simulink model "JenaFox_moodle_ISB"  (R2018a)
settings: Solver=ode23s  StartTime=0.0  StopTime=60  MaxStep=maxStep  RelTol=relTol  AbsTol=absTol
InitFcn:
  | Fox_param;
model workspace: external: MAT-File C:\Users\Work\Documents\MATLAB\JenaFoxSimulink\moodle model\simulink_robot_DataFile.mat (data not in the file)
undefined symbols (not defined in the file or in its folder): amplifier, c_coupling_hip, c_coupling_knee, c_hs, d_coupling_knee, d_hs, g, hip_i, hip_Jm, hip_k, hip_Mrg, hip_Mrhg, hip_na, hip_Ra, IC_motor_hip_l, IC_motor_hip_r, IC_motor_knee_l, IC_motor_knee_r, IC_phi_hip_l, IC_phi_hip_r, IC_v_motor_hip, IC_v_motor_knee, k_gx, k_gy, knee_i, knee_Jm, knee_k, knee_Mrg, knee_Mrhg, knee_na, knee_Ra, mu_slide, mu_stick, smiData, v_gx_max, v_gy_max, vLimit, X, Y, Z
libraries: sm_lib x38, nesl_utility x28, simulink x22, simulink_extras x8
(part 3 of 3)

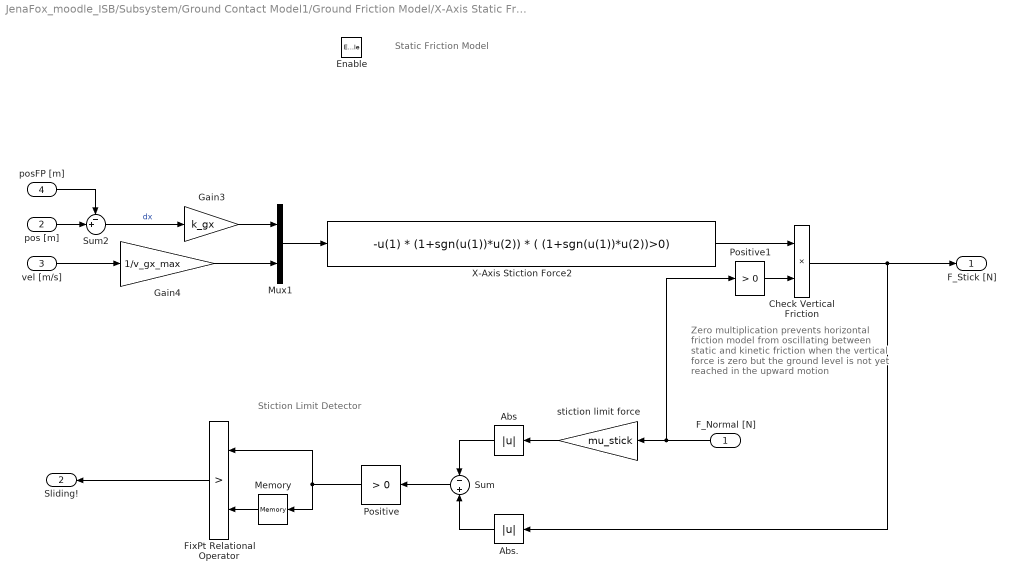
== system JenaFox_moodle_ISB/Subsystem/Ground Contact Model1/Ground Friction Model/X-Axis Static Friction Model ==
  note: Stiction Limit Detector
  note: Static Friction Model
  note: Zero multiplication prevents
      | horizontal friction model from
      | oscillating between static and kinetic
      | friction when the vertical force is zero but
      | the ground level is not yet reached
      | in the upward motion
  F_Normal [N] : Inport
  pos [m] : Inport  Port=2
  vel [m/s] : Inport  Port=3
  posFP [m] : Inport  Port=4
  Enable : EnablePort  StatesWhenEnabling=reset  PropagateVarSize=During execution
  Abs : Abs
  Abs. : Abs
  Check Vertical Friction : Product  RndMeth=Zero
  FixPt Relational Operator : RelationalOperator  Operator=>  OutDataTypeStr=boolean  ZeroCross=off  RndMeth=Nearest
  Gain3 : Gain  Gain=k_gx
  Gain4 : Gain  Gain=1/v_gx_max
  Memory : Memory
  Mux1 : Mux  Inputs=2
  Positive : simulink/Logic and Bit Operations/Compare To Zero  relop=>  OutDataTypeStr=boolean
  Positive1 : simulink/Logic and Bit Operations/Compare To Zero  relop=>  OutDataTypeStr=boolean
  Sum : Sum  Inputs=-+
  Sum2 : Sum  Inputs=-+|
  X-Axis Stiction Force2 : Fcn  Expr=-u(1) * (1+sgn(u(1))*u(2)) * ( (1+sgn(u(1))*u(2))>0)
  stiction limit force : Gain  Gain=mu_stick
  F_Stick [N] : Outport  OutputWhenDisabled=reset  InitialOutput=0
      settings: AttributesFormatString=when disabled: %<OutputWhenDisabled>\ninitial: %<InitialOutput>
  Sliding! : Outport  Port=2  OutputWhenDisabled=reset  InitialOutput=0
      settings: AttributesFormatString=when disabled: %<OutputWhenDisabled>\ninitial: %<InitialOutput>
  wires:
  F_Normal [N]/1 -> stiction limit force/1, Positive1/1
  Sum2/1 -> Gain3/1  "dx"
  pos [m]/1 -> Sum2/2
  posFP [m]/1 -> Sum2/1
  vel [m/s]/1 -> Gain4/1
  Sum/1 -> Positive/1
  Memory/1 -> FixPt Relational Operator/2
  Positive/1 -> FixPt Relational Operator/1, Memory/1
  Abs./1 -> Sum/2
  Mux1/1 -> X-Axis Stiction Force2/1
  Gain3/1 -> Mux1/1
  Gain4/1 -> Mux1/2
  FixPt Relational Operator/1 -> Sliding!/1
  Abs/1 -> Sum/1
  stiction limit force/1 -> Abs/1
  Positive1/1 -> Check Vertical Friction/2
  Check Vertical Friction/1 -> F_Stick [N]/1, Abs./1
  X-Axis Stiction Force2/1 -> Check Vertical Friction/1

== system JenaFox_moodle_ISB/Subsystem/simulation terminator/Subsystem/Subsystem ==
  In1 : Inport
  Enable : EnablePort  StatesWhenEnabling=reset
  Compare To Constant5 : simulink/Logic and Bit Operations/Compare To Constant  relop=>=  const=5  OutDataTypeStr=boolean
  Out1 : Outport
  wires:
  Compare To Constant5/1 -> Out1/1
  In1/1 -> Compare To Constant5/1

== matlab function JenaFox_moodle_ISB/neural network for torque control ==
  data: t_0 input; phi input; GC input; y_latched input size=8; t_1 input; U output size=4; t_0 output; y output size=8
function [U, t_0, y]  = neuro_control(t_0,phi,GC, y_latched, t_1)
% calculates the motor torques for the runbot model with a neural network
% (method described in Geng 2006 IEEE Trans. Mech.

% GC Ground Contact for right foot and left foot
rho_GR = GC(1);
rho_GL = GC(2);

% phi is the angle hip_r, hip_l, knee_r and knee_l
phi_hip_r = phi(1);
phi_hip_l = phi(2);
phi_knee_r = phi(3);
phi_knee_l = phi(4);

%% Time tracking
if isempty(t_0)
    t_0 =0;
end
delta_t = t_1-t_0; 
t_0 = t_1;

%% Define Sensor Neurons
% Activation threshold for the sensor neurons
theta_eh = 5; 
theta_fh = -10;
theta_ek = -3;
theta_fk = -80;

% Activation threshold for the stretch receptors
theta_AL = theta_fh; 
theta_AR = theta_fh; 

% Positive constant for the exponential 
alpha_AL = 2;
alpha_AR = 2;
alpha_h = 2;
alpha_k = 2;

% The activation functions for the sensor neurons AL and AR
rho_AL = 1/(1+exp(alpha_AL*-(theta_AL-phi_hip_l)));
rho_AR = 1/(1+exp(alpha_AR*-(theta_AR-phi_hip_r)));

% The activation functions for the sensor neurons in the joints
% The Right Hip
rho_es_rh = 1 / (1+exp(alpha_h*(theta_eh - phi_hip_r)));
rho_fs_rh = 1 / (1+exp(alpha_h*(phi_hip_r - theta_fh)));
% The Left Hip
rho_es_lh = 1/(1+exp(alpha_h*(theta_eh - phi_hip_l)));
rho_fs_lh = 1/(1+exp(alpha_h*(phi_hip_l - theta_fh)));
% The Right Knee
rho_es_rk = 1/(1+exp(alpha_k*(theta_ek - phi_knee_r)));
rho_fs_rk = 1/(1+exp(alpha_k*(phi_knee_r - theta_fk)));
% The Left Knee
rho_es_lk = 1/(1+exp(alpha_k*(theta_ek - phi_knee_l)));
rho_fs_lk = 1/(1+exp(alpha_k*(phi_knee_l - theta_fk)));


%% Define the Motor Neurons
% Input for motor neurons
if isempty(y_latched)
    y_latched=zeros(8,1);
end
y=zeros(8,1);

% Motor voltage output
U = zeros(4,1); % 1 right hip, 2 left hip, 3 right knee, 4 left knee

% Capacitor voltage R = 1kOhm, C = 10uF
tau     = 1e3*10e-6;
GM_h    = 1.5;
GM_k    = 0.9*GM_h;
M_amp   = 3;

% Threshold for the sigmoid activation function
theta_m = 1;

% The impulse response for the motor neurons:
% u = u_0exp(-t/RC) + sum(w_i + rho_i)

% The Right Hip
sum_em_rh = -30*rho_es_rh + 10*rho_GR - 10*rho_GL;
y(1) = y_latched(1)*exp(-delta_t/tau) + sum_em_rh;
u_rh_e = 1/(1 + exp(theta_m-y(1)));
sum_fm_rh = -30*rho_fs_rh + 10*rho_GL - 10*rho_GR;
y(2) = y_latched(2)*exp(-delta_t/tau) + sum_fm_rh;
u_rh_f = 1/(1 + exp(theta_m-y(2)));
U(1) = M_amp*GM_h*(u_rh_e - u_rh_f);

% The Left Hip
sum_em_lh = -30*rho_es_lh + 10*rho_GL - 10*rho_GR;
y(3) = y_latched(3)*exp(-delta_t/tau) + sum_em_lh;
u_lh_e = 1/(1 + exp(theta_m-y(3)));
sum_fm_lh = -30*rho_fs_lh + 10*rho_GR - 10*rho_GL;
y(4) = y_latched(4)*exp(-delta_t/tau) + sum_fm_lh;
u_lh_f = 1/(1 + exp(theta_m-y(4)));
U(2) = M_amp*GM_h*(u_lh_e - u_lh_f);

% The Right Knee
sum_em_rk = -30*rho_es_rk - 10*rho_GL + 10*rho_GR + 15*rho_AR;
y(5) = y_latched(5)*exp(-delta_t/tau) + sum_em_rk;
u_rk_e = 1/(1 + exp(theta_m-y(5)));
sum_fm_rk = -30*rho_fs_rk - 10*rho_GR + 10*rho_GL - 15*rho_AR;
y(6) = y_latched(6)*exp(-delta_t/tau) + sum_fm_rk;
u_rk_f = 1/(1 + exp(theta_m-y(6)));
U(3) = M_amp*GM_k*(u_rk_e - u_rk_f);

% The Left Knee
sum_em_lk = -30*rho_es_lk - 10*rho_GR + 10*rho_GL + 15*rho_AL;
y(7) = y_latched(7)*exp(-delta_t/tau) + sum_em_lk;
u_lk_e = 1/(1 + exp(theta_m-y(7)));
sum_fm_lk = -30*rho_fs_lk - 10*rho_GL + 10*rho_GR - 15*rho_AL;
y(8) = y_latched(8)*exp(-delta_t/tau) + sum_fm_lk;
u_lk_f = 1/(1 + exp(theta_m-y(8)));
U(4) = M_amp*GM_k*(u_lk_e - u_lk_f);



end
